simulink model "WaermeflussSchaltschrank_V1"  (Simulink 7.6)
settings: Solver=ode45  StartTime=0.0  StopTime=SimulTime  RelTol=1e-3
values from neighbouring files (symbols this model uses):
  Anzahl = 2    [ParametersWaermeflussSchaltschrank.m]
  EinRittal = 1    [ParametersWaermeflussSchaltschrank.m]
  f1 = 0.3448    [ParametersWaermeflussSchaltschrank.m]
  geometrie = l+l1    (= 4.01318327974)    [ParametersWaermeflussSchaltschrank.m]
  P_Rittal = 1200    [ParametersWaermeflussSchaltschrank.m]
  P_SA = 60000    [ParametersWaermeflussSchaltschrank.m]
  Pr = 0.7    [ParametersWaermeflussSchaltschrank.m]
  sb = 5.67*(10^-8)    (= 5.67e-08)    [ParametersWaermeflussSchaltschrank.m]
  T_Umgebung = 296    [ParametersWaermeflussSchaltschrank.m]
  VentilatorRittal = 80    [ParametersWaermeflussSchaltschrank.m]
undefined symbols (not defined in the file or in its folder): A, CNC, KinematischeViskositaet, n, Schaltschrank_Kuehlung, Temperatur, Waermeleitfaehigkeit
settings Model: Creator=conid  LastModifiedBy=conid

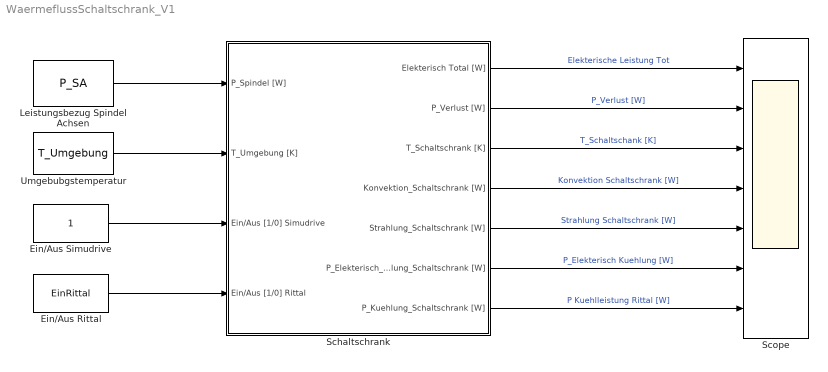
== system WaermeflussSchaltschrank_V1 ==
  Ein/Aus Rittal : Constant  Value=EinRittal
  Ein/Aus Simudrive : Constant
  Leistungsbezug Spindel Achsen : Constant  Value=P_SA
  Schaltschrank : Subsystem  TreatAsAtomicUnit=on
  Scope : Scope  NumInputPorts=7
      settings: YMin=-5~-5~-5~-5~-5~-5~-5  YMax=5~5~5~5~5~5~5  SaveName=Scp_Cabinet
  Umgebubgstemperatur : Constant  Value=T_Umgebung
  wires:
  Schaltschrank/1(Elekterisch Total [W]) -> Scope/1  "Elekterische Leistung Tot"
  Schaltschrank/3(T_Schaltschrank [K]) -> Scope/3  "T_Schaltschank [K]"
  Schaltschrank/4(Konvektion_Schaltschrank [W]) -> Scope/4  "Konvektion Schaltschrank [W]"
  Schaltschrank/5(Strahlung_Schaltschrank [W]) -> Scope/5  "Strahlung Schaltschrank [W]"
  Schaltschrank/6(P_Elekterisch_Kuehlung_Schaltschrank [W]) -> Scope/6  "P_Elekterisch Kuehlung [W]"
  Schaltschrank/7(P_Kuehlung_Schaltschrank [W]) -> Scope/7  "P Kuehlleistung Rittal [W]"
  Leistungsbezug Spindel Achsen/1 -> Schaltschrank/1(P_Spindel [W])
  Umgebubgstemperatur/1 -> Schaltschrank/2(T_Umgebung [K])
  Ein/Aus Simudrive/1 -> Schaltschrank/3(Ein/Aus [1/0] Simudrive)
  Schaltschrank/2(P_Verlust [W]) -> Scope/2  "P_Verlust [W]"
  Ein/Aus Rittal/1 -> Schaltschrank/4(Ein/Aus [1/0] Rittal)

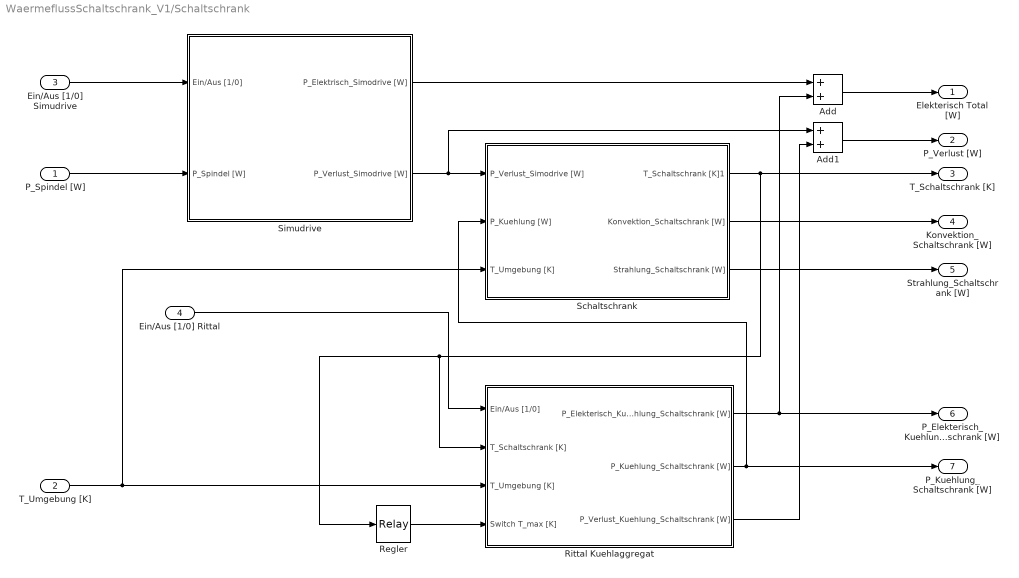
== system WaermeflussSchaltschrank_V1/Schaltschrank ==
  P_Spindel [W] : Inport
  T_Umgebung [K] : Inport  Port=2
  Ein/Aus [1/0] Simudrive : Inport  Port=3
  Ein/Aus [1/0] Rittal : Inport  Port=4
  Add : Sum
  Add1 : Sum
  Regler : Relay  OnSwitchValue=Schaltschrank_Kuehlung.Tmax  OffSwitchValue=Schaltschrank_Kuehlung.Tmin
  Rittal Kuehlaggregat : Subsystem
  Schaltschrank : Subsystem
  Simudrive : Subsystem
  Elekterisch Total [W] : Outport
  P_Verlust [W] : Outport  Port=2
  T_Schaltschrank [K] : Outport  Port=3
  Konvektion_Schaltschrank [W] : Outport  Port=4
  Strahlung_Schaltschrank [W] : Outport  Port=5
  P_Elekterisch_Kuehlung_Schaltschrank [W] : Outport  Port=6
  P_Kuehlung_Schaltschrank [W] : Outport  Port=7
  wires:
  Schaltschrank/1(T_Schaltschrank [K]1) -> Regler/1, Rittal Kuehlaggregat/2(T_Schaltschrank [K]), T_Schaltschrank [K]/1
  T_Umgebung [K]/1 -> Rittal Kuehlaggregat/3(T_Umgebung [K]), Schaltschrank/3(T_Umgebung [K])
  Rittal Kuehlaggregat/2(P_Kuehlung_Schaltschrank [W]) -> Schaltschrank/2(P_Kuehlung [W]), P_Kuehlung_Schaltschrank [W]/1
  Schaltschrank/2(Konvektion_Schaltschrank [W]) -> Konvektion_Schaltschrank [W]/1
  Schaltschrank/3(Strahlung_Schaltschrank [W]) -> Strahlung_Schaltschrank [W]/1
  Rittal Kuehlaggregat/1(P_Elekterisch_Kuehlung_Schaltschrank [W]) -> P_Elekterisch_Kuehlung_Schaltschrank [W]/1, Add/2
  P_Spindel [W]/1 -> Simudrive/2(P_Spindel [W])
  Ein/Aus [1/0] Simudrive/1 -> Simudrive/1(Ein/Aus [1/0])
  Simudrive/2(P_Verlust_Simodrive [W]) -> Schaltschrank/1(P_Verlust_Simodrive [W]), Add1/1
  Simudrive/1(P_Elektrisch_Simodrive [W]) -> Add/1
  Regler/1 -> Rittal Kuehlaggregat/4(Switch T_max [K])
  Add/1 -> Elekterisch Total [W]/1
  Rittal Kuehlaggregat/3(P_Verlust_Kuehlung_Schaltschrank [W]) -> Add1/2
  Add1/1 -> P_Verlust [W]/1
  Ein/Aus [1/0] Rittal/1 -> Rittal Kuehlaggregat/1(Ein/Aus [1/0])

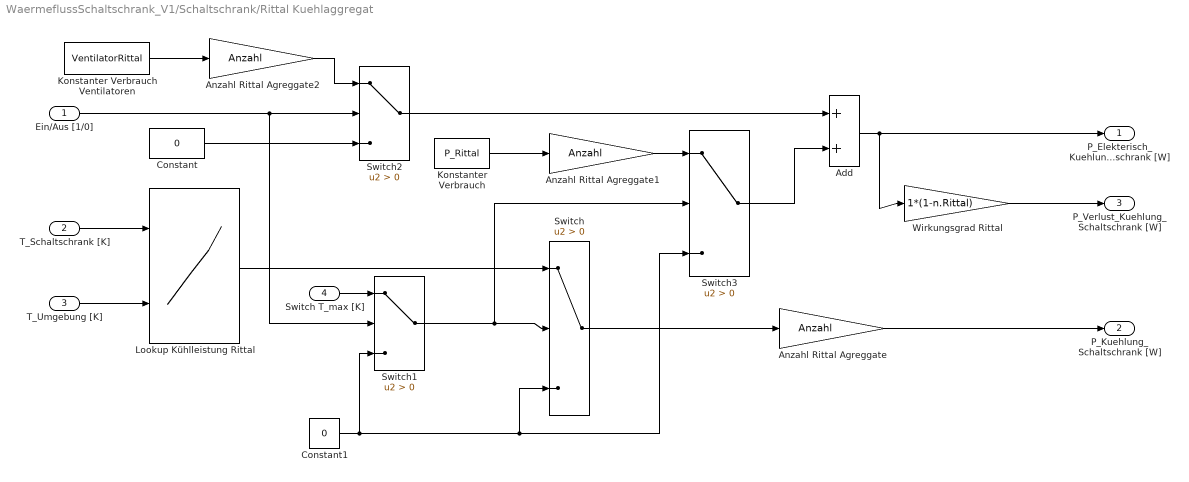
== system WaermeflussSchaltschrank_V1/Schaltschrank/Rittal Kuehlaggregat ==
  Ein/Aus [1/0] : Inport
  T_Schaltschrank [K] : Inport  Port=2
  T_Umgebung [K] : Inport  Port=3
  Switch T_max [K] : Inport  Port=4
  Add : Sum
  Anzahl Rittal Agreggate : Gain  Gain=Anzahl
  Anzahl Rittal Agreggate1 : Gain  Gain=Anzahl
  Anzahl Rittal Agreggate2 : Gain  Gain=Anzahl
  Constant : Constant  Value=0
  Constant1 : Constant  Value=0
  "Konstanter Verbrauch " : Constant  Value=P_Rittal
  Konstanter Verbrauch Ventilatoren : Constant  Value=VentilatorRittal
  Lookup Kühlleistung Rittal : Lookup_n-D  BreakpointsForDimension1=Schaltschrank_Kuehlung.T_int  BreakpointsForDimension2=Schaltschrank_Kuehlung.T_ext  Table=Schaltschrank_Kuehlung.Qdot  InterpMethod=Cubic spline  ExtrapMethod=None - Clip  InputSameDT=on
  Switch{,1..3} (4 alike) : Switch  Criteria=u2 > Threshold
  Wirkungsgrad Rittal : Gain  Gain=1*(1-n.Rittal)
  P_Elekterisch_Kuehlung_Schaltschrank [W] : Outport
  P_Kuehlung_Schaltschrank [W] : Outport  Port=2
  P_Verlust_Kuehlung_Schaltschrank [W] : Outport  Port=3
  wires:
  Lookup Kühlleistung Rittal/1 -> Switch/1
  Ein/Aus [1/0]/1 -> Switch2/2, Switch1/2
  Constant/1 -> Switch2/3
  Switch2/1 -> Add/1
  Add/1 -> P_Elekterisch_Kuehlung_Schaltschrank [W]/1, Wirkungsgrad Rittal/1
  Constant1/1 -> Switch/3, Switch3/3, Switch1/3
  T_Umgebung [K]/1 -> Lookup Kühlleistung Rittal/2
  T_Schaltschrank [K]/1 -> Lookup Kühlleistung Rittal/1
  Switch3/1 -> Add/2
  Anzahl Rittal Agreggate/1 -> P_Kuehlung_Schaltschrank [W]/1
  Switch/1 -> Anzahl Rittal Agreggate/1
  Wirkungsgrad Rittal/1 -> P_Verlust_Kuehlung_Schaltschrank [W]/1
  Switch1/1 -> Switch/2, Switch3/2
  Switch T_max [K]/1 -> Switch1/1
  Anzahl Rittal Agreggate1/1 -> Switch3/1
  "Konstanter Verbrauch "/1 -> Anzahl Rittal Agreggate1/1
  Anzahl Rittal Agreggate2/1 -> Switch2/1
  Konstanter Verbrauch Ventilatoren/1 -> Anzahl Rittal Agreggate2/1

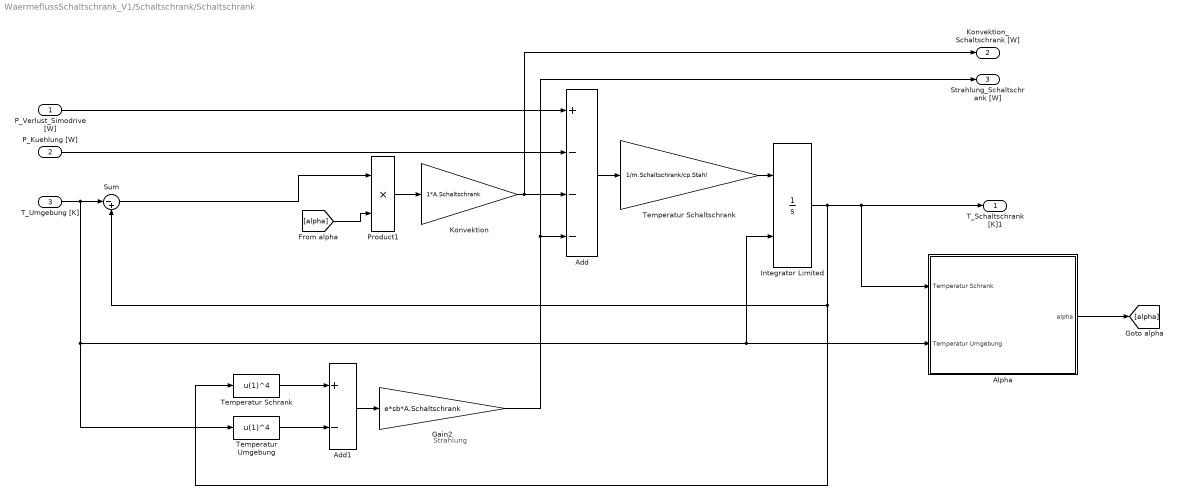
== system WaermeflussSchaltschrank_V1/Schaltschrank/Schaltschrank ==
  note: Strahlung
  P_Verlust_Simodrive [W] : Inport
  P_Kuehlung [W] : Inport  Port=2
  T_Umgebung [K] : Inport  Port=3
  Add : Sum  Inputs=+---
  Add1 : Sum  Inputs=+-
  Alpha : Subsystem
  Gain2 : Gain  Gain=e*sb*A.Schaltschrank
  Integrator Limited : Integrator  InitialConditionSource=external  LimitOutput=on
  Konvektion : Gain  Gain=1*A.Schaltschrank
  Product1 : Product  RndMeth=Zero
  Sum : Sum  Inputs=|-+
  Temperatur Schaltschrank : Gain  Gain=1/m.Schaltschrank/cp.Stahl
  Temperatur Schrank : Fcn  Expr=u(1)^4
  Temperatur Umgebung : Fcn  Expr=u(1)^4
  T_Schaltschrank [K]1 : Outport
  Konvektion_Schaltschrank [W] : Outport  Port=2
  Strahlung_Schaltschrank [W] : Outport  Port=3
  wires:
  P_Verlust_Simodrive [W]/1 -> Add/1
  Temperatur Schaltschrank/1 -> Integrator Limited/1
  Integrator Limited/1 -> T_Schaltschrank [K]1/1, Alpha/1(Temperatur Schrank), Sum/2, Temperatur Schrank/1
  Add/1 -> Temperatur Schaltschrank/1
  Gain2/1 -> Strahlung_Schaltschrank [W]/1, Add/4
  P_Kuehlung [W]/1 -> Add/2
  Add1/1 -> Gain2/1
  Temperatur Schrank/1 -> Add1/1
  Sum/1 -> Product1/1
  T_Umgebung [K]/1 -> Sum/1, Integrator Limited/2, Alpha/2(Temperatur Umgebung), Temperatur Umgebung/1
  Temperatur Umgebung/1 -> Add1/2
  Product1/1 -> Konvektion/1
  [alpha] -> Product1/2
  Konvektion/1 -> Add/3, Konvektion_Schaltschrank [W]/1
  Alpha/1(alpha) -> [alpha]

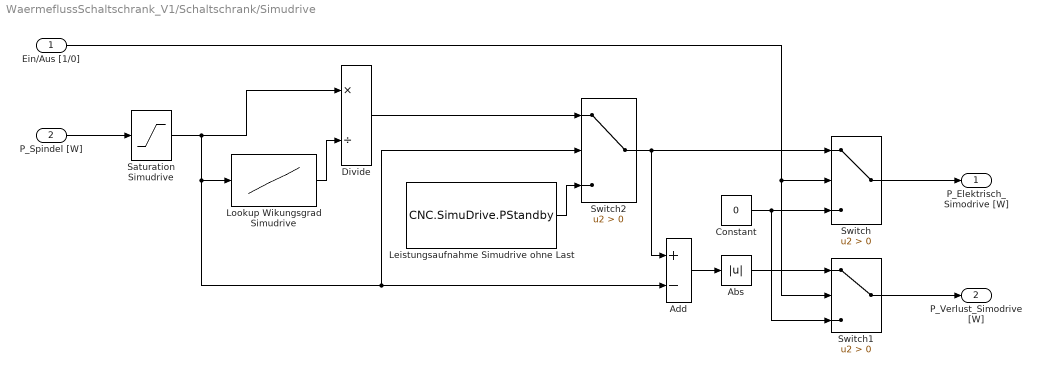
== system WaermeflussSchaltschrank_V1/Schaltschrank/Simudrive ==
  Ein/Aus [1/0] : Inport
  P_Spindel [W] : Inport  Port=2
  Abs : Abs
  Add : Sum  Inputs=+-
  Constant : Constant  Value=0
  Divide : Product  Inputs=*/
  Leistungsaufnahme Simudrive ohne Last : Constant  Value=CNC.SimuDrive.PStandby
  Lookup Wikungsgrad Simudrive : Lookup_n-D  NumberOfTableDimensions=1  BreakpointsForDimension1=CNC.SimuDrive.OpPointsP  Table=CNC.SimuDrive.OpPointsEta  InputSameDT=on
  Saturation Simudrive : Saturate  UpperLimit=CNC.SimuDrive.MaxP  LowerLimit=-CNC.SimuDrive.MaxP
  Switch : Switch  Criteria=u2 > Threshold
  Switch1 : Switch  Criteria=u2 > Threshold
  Switch2 : Switch  Criteria=u2 > Threshold
  P_Elektrisch_Simodrive [W] : Outport
  P_Verlust_Simodrive [W] : Outport  Port=2
  wires:
  Switch1/1 -> P_Verlust_Simodrive [W]/1
  Switch/1 -> P_Elektrisch_Simodrive [W]/1
  Abs/1 -> Switch1/1
  Constant/1 -> Switch/3, Switch1/3
  Add/1 -> Abs/1
  Switch2/1 -> Switch/1, Add/1
  P_Spindel [W]/1 -> Saturation Simudrive/1
  Lookup Wikungsgrad Simudrive/1 -> Divide/2
  Divide/1 -> Switch2/1
  Leistungsaufnahme Simudrive ohne Last/1 -> Switch2/3
  Saturation Simudrive/1 -> Divide/1, Add/2, Switch2/2, Lookup Wikungsgrad Simudrive/1
  Ein/Aus [1/0]/1 -> Switch/2, Switch1/2

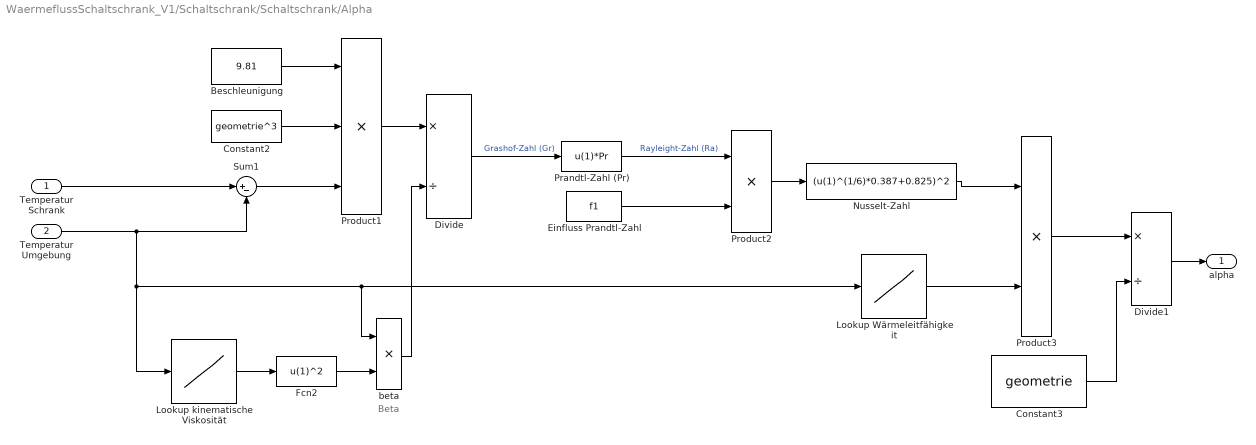
== system WaermeflussSchaltschrank_V1/Schaltschrank/Schaltschrank/Alpha ==
  note: Beta
  Temperatur Schrank : Inport
  Temperatur Umgebung : Inport  Port=2
  Beschleunigung : Constant  Value=9.81
  Constant2 : Constant  Value=geometrie^3
  Constant3 : Constant  Value=geometrie
  Divide : Product  Inputs=*/
  Divide1 : Product  Inputs=*/
  Einfluss Prandtl-Zahl : Constant  Value=f1
  Fcn2 : Fcn  Expr=u(1)^2
  Lookup Wärmeleitfähigkeit : Lookup_n-D  NumberOfTableDimensions=1  BreakpointsForDimension1=Temperatur.Tabel  Table=Waermeleitfaehigkeit.Tabel  InterpMethod=Cubic spline  ExtrapMethod=None - Clip  InputSameDT=on
  Lookup kinematische Viskosität : Lookup_n-D  NumberOfTableDimensions=1  BreakpointsForDimension1=Temperatur.Tabel  Table=KinematischeViskositaet.Tabel  InterpMethod=Cubic spline  ExtrapMethod=None - Clip  InputSameDT=on
  Nusselt-Zahl : Fcn  Expr=(u(1)^(1/6)*0.387+0.825)^2
  Prandtl-Zahl (Pr) : Fcn  Expr=u(1)*Pr
  Product1 : Product  Inputs=3  RndMeth=Zero
  Product2 : Product  RndMeth=Zero
  Product3 : Product  RndMeth=Zero
  Sum1 : Sum  Inputs=|+-
  beta : Product  RndMeth=Zero
  alpha : Outport
  wires:
  Sum1/1 -> Product1/3
  Constant2/1 -> Product1/2
  Beschleunigung/1 -> Product1/1
  Product1/1 -> Divide/1
  Divide/1 -> Prandtl-Zahl (Pr)/1  "Grashof-Zahl (Gr)"
  Prandtl-Zahl (Pr)/1 -> Product2/1  "Rayleight-Zahl (Ra)"
  Einfluss Prandtl-Zahl/1 -> Product2/2
  Product2/1 -> Nusselt-Zahl/1
  Nusselt-Zahl/1 -> Product3/1
  Lookup Wärmeleitfähigkeit/1 -> Product3/2
  Product3/1 -> Divide1/1
  Constant3/1 -> Divide1/2
  Divide1/1 -> alpha/1
  Lookup kinematische Viskosität/1 -> Fcn2/1
  Fcn2/1 -> beta/2
  beta/1 -> Divide/2
  Temperatur Schrank/1 -> Sum1/1
  Temperatur Umgebung/1 -> Sum1/2, Lookup kinematische Viskosität/1, beta/1, Lookup Wärmeleitfähigkeit/1
